simulink model "CheckoutLines"  (R2020a)
settings: Solver=VariableStepAuto  StartTime=0.0  StopTime=14400  RelTol=1e-3
undefined symbols (not defined in the file): m, n
libraries: dspstat3 x2
settings Model: Creator=jggam  LastModifiedBy=jggam

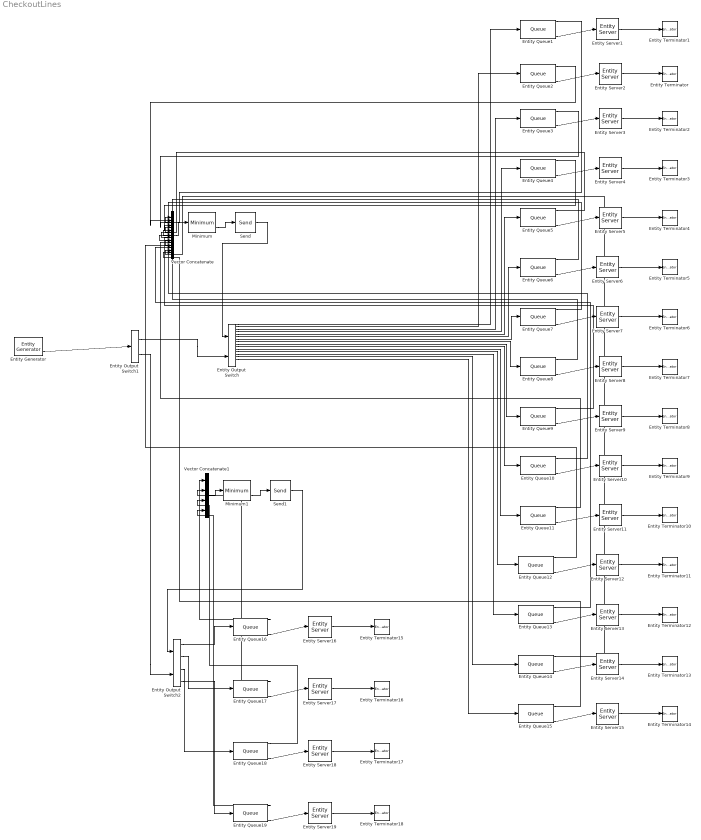
== system CheckoutLines ==
  Entity Output Switch : EntityOutputSwitch  InputPortMessageModes=m,m  OutputPortMessageModes=m,m,m,m,m,m,m,m,m,m,m,m,m,m,m,m,m,m  NumberOutputPorts=18  SwitchingCriterion=From control port  SwitchAttributeName=Attribute1
      settings: InputPortMap=u0,u1  OutputPortMap=o0,o1,o2,o3,o4,o5,o6,o7,o8,o9,o10,o11,o12,o13,o14,o15,o16,o17
  Entity Output Switch1 : EntityOutputSwitch  InputPortMessageModes=m  OutputPortMessageModes=m,m  SwitchingCriterion=From attribute  SwitchAttributeName=noExpress
  Entity Output Switch2 : EntityOutputSwitch  InputPortMessageModes=m,m  OutputPortMessageModes=m,m,m,m  NumberOutputPorts=4  SwitchingCriterion=From control port  SwitchAttributeName=Attribute1
      settings: InputPortMap=u0,u1  OutputPortMap=o0,o1,o2,o3
  Entity Generator : EntityGenerator  OutputPortMessageModes=n,m  TimeSource=MATLAB action  Period=0.5  IntergenerationTimeAction=dt = arrivalTime(RandArrivalTimesDist);  GenerateEntityAtSimulationStart=off  GenerateAction=|  AttributeName=NumberOfItems|ServiceTime|row|expressEligible|noExpress  AttributeInitialValue=1|1|1|1|1  NumberEntitiesDeparted=on  EntityType=Structured  EntityTypeName=Entity
      | entity.row = randrow(AllCheckouts);
      | entity.NumberOfItems = numberOfItems(AllCheckouts,entity.row);
      | entity.ServiceTime = serviceTime(AllCheckouts,entity.row);
      | if entity.NumberOfItems <= 10
      |     entity.expressEligible = 2;
      | end
      settings: OutputPortMap=o0,o3
  Entity Queue{1..19} (19 alike) : Queue  InputPortMessageModes=m  OutputPortMessageModes=n,n,n,m  Capacity=QueueCapacity  NumberEntitiesInBlock=on  AverageWait=on  AverageQueueLength=on
      settings: OutputPortMap=o1,o2,o3,o5
  Entity Server{1..19} (19 alike) : EntityServer  InputPortMessageModes=m  OutputPortMessageModes=m  Capacity=1  ServiceTimeSource=MATLAB action  ServiceTimeValue=1.75  ServiceTimeAction=dt = entity.ServiceTime;
  Entity Terminator{,1..18} (19 alike) : EntityTerminator  InputPortMessageModes=m
  Minimum : dspstat3/Minimum  operation=minimum  fcn=Value and Index  indexBase=One  operateOver=Entire input  Dimension=1  InputProcessing=Columns as channels (frame based)  reset=None  roiEnable=off  roiType=Rectangles  roiPortion=Entire ROI  roiOutput=Individual statistics for each ROI  roiFlag=off  roundingMode=Floor  overflowMode=off
      settings: SourceProductBaseCode=DS
  Minimum1 : dspstat3/Minimum  operation=minimum  fcn=Value and Index  indexBase=One  operateOver=Entire input  Dimension=1  InputProcessing=Columns as channels (frame based)  reset=None  roiEnable=off  roiType=Rectangles  roiPortion=Entire ROI  roiOutput=Individual statistics for each ROI  roiFlag=off  roundingMode=Floor  overflowMode=off
      settings: SourceProductBaseCode=DS
  Send : Send  OutputPortMessageModes=m
  Send1 : Send  OutputPortMessageModes=m
  Vector Concatenate : Concatenate  NumInputs=15
  Vector Concatenate1 : Concatenate  NumInputs=4
  wires:
  Entity Queue1/4 -> Entity Server1/1
  Entity Queue2/4 -> Entity Server2/1
  Entity Queue3/4 -> Entity Server3/1
  Entity Output Switch/2 -> Entity Queue2/1
  Entity Output Switch/1 -> Entity Queue1/1
  Entity Output Switch/3 -> Entity Queue3/1
  Entity Queue1/1 -> Vector Concatenate/1
  Entity Queue2/1 -> Vector Concatenate/2
  Entity Queue3/1 -> Vector Concatenate/3
  Vector Concatenate/1 -> Minimum/1
  Entity Server2/1 -> Entity Terminator/1
  Entity Server1/1 -> Entity Terminator1/1
  Send/1 -> Entity Output Switch/1
  Entity Server3/1 -> Entity Terminator2/1
  Entity Queue7/4 -> Entity Server7/1
  Entity Queue6/4 -> Entity Server6/1
  Entity Queue5/4 -> Entity Server5/1
  Entity Queue4/4 -> Entity Server4/1
  Entity Server4/1 -> Entity Terminator3/1
  Entity Server5/1 -> Entity Terminator4/1
  Entity Server6/1 -> Entity Terminator5/1
  Entity Server7/1 -> Entity Terminator6/1
  Entity Output Switch/4 -> Entity Queue4/1
  Entity Output Switch/5 -> Entity Queue5/1
  Entity Output Switch/6 -> Entity Queue6/1
  Entity Queue4/1 -> Vector Concatenate/4
  Entity Queue5/1 -> Vector Concatenate/5
  Entity Queue6/1 -> Vector Concatenate/6
  Entity Queue7/1 -> Vector Concatenate/7
  Entity Queue10/4 -> Entity Server10/1
  Entity Queue9/4 -> Entity Server9/1
  Entity Server8/1 -> Entity Terminator7/1
  Entity Server9/1 -> Entity Terminator8/1
  Entity Queue8/4 -> Entity Server8/1
  Entity Queue10/1 -> Vector Concatenate/10
  Entity Output Switch/7 -> Entity Queue7/1
  Entity Output Switch/8 -> Entity Queue8/1
  Entity Output Switch/10 -> Entity Queue10/1
  Entity Output Switch/9 -> Entity Queue9/1
  Entity Queue8/1 -> Vector Concatenate/8
  Entity Queue9/1 -> Vector Concatenate/9
  Entity Queue11/4 -> Entity Server11/1
  Entity Server11/1 -> Entity Terminator10/1
  Entity Queue12/4 -> Entity Server12/1
  Entity Server12/1 -> Entity Terminator11/1
  Entity Queue13/4 -> Entity Server13/1
  Entity Server13/1 -> Entity Terminator12/1
  Entity Queue14/4 -> Entity Server14/1
  Entity Server14/1 -> Entity Terminator13/1
  Entity Output Switch/11 -> Entity Queue11/1
  Entity Queue11/1 -> Vector Concatenate/11
  Entity Output Switch/12 -> Entity Queue12/1
  Entity Server10/1 -> Entity Terminator9/1
  Entity Output Switch/13 -> Entity Queue13/1
  Entity Output Switch/14 -> Entity Queue14/1
  Entity Queue13/1 -> Vector Concatenate/13
  Entity Queue14/1 -> Vector Concatenate/14
  Entity Queue16/4 -> Entity Server16/1
  Entity Server16/1 -> Entity Terminator15/1
  Entity Queue17/4 -> Entity Server17/1
  Entity Server17/1 -> Entity Terminator16/1
  Entity Queue18/4 -> Entity Server18/1
  Entity Server18/1 -> Entity Terminator17/1
  Entity Output Switch1/2 -> Entity Output Switch2/2
  Entity Server19/1 -> Entity Terminator18/1
  Entity Queue19/4 -> Entity Server19/1
  Entity Queue16/1 -> Vector Concatenate1/1
  Entity Queue17/1 -> Vector Concatenate1/2
  Entity Queue18/1 -> Vector Concatenate1/3
  Entity Queue19/1 -> Vector Concatenate1/4
  Entity Output Switch2/1 -> Entity Queue16/1
  Entity Output Switch2/2 -> Entity Queue17/1
  Entity Output Switch2/3 -> Entity Queue18/1
  Entity Output Switch2/4 -> Entity Queue19/1
  Vector Concatenate1/1 -> Minimum1/1
  Minimum1/2 -> Send1/1
  Send1/1 -> Entity Output Switch2/1
  Entity Generator/2 -> Entity Output Switch1/1
  Entity Output Switch1/1 -> Entity Output Switch/2
  Entity Queue12/1 -> Vector Concatenate/12
  Entity Queue15/4 -> Entity Server15/1
  Entity Server15/1 -> Entity Terminator14/1
  Entity Output Switch/15 -> Entity Queue15/1
  Entity Queue15/1 -> Vector Concatenate/15
  Minimum/2 -> Send/1
